simulink model "Wahsing_Mashine_1650800329"  (R2021a)
settings: Solver=VariableStepAuto  StartTime=0.0  StopTime=500  RelTol=1e-3
settings Model: Creator=Ish  LastModifiedBy=Ish

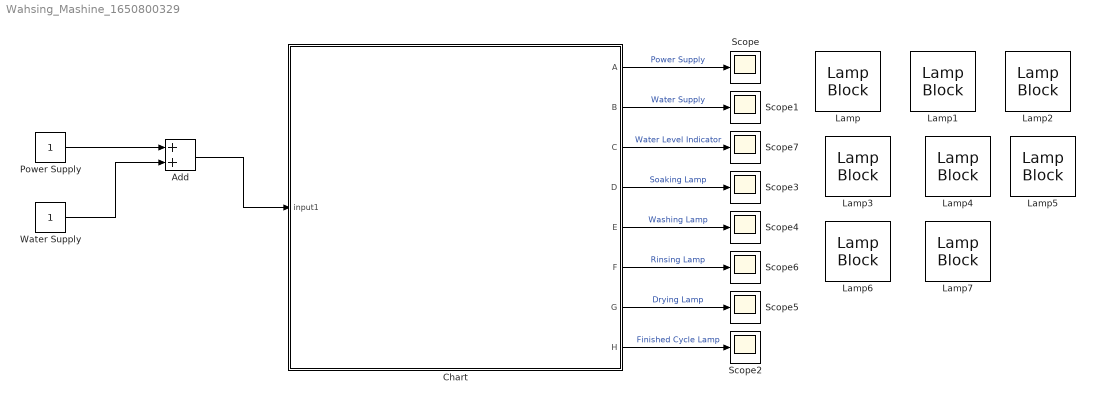
== system Wahsing_Mashine_1650800329 ==
  Add : Sum
  Chart : Stateflow chart  TreatAsAtomicUnit=on
  Lamp{,1..7} (8 alike) : LampBlock  Icon=Circle
  Power Supply : Constant
  Scope{,1..7} (8 alike) : Scope
  Water Supply : Constant
  wires:
  Water Supply/1 -> Add/2
  Power Supply/1 -> Add/1
  Add/1 -> Chart/1(input1)
  Chart/1(A) -> Scope/1  "Power Supply"
  Chart/2(B) -> Scope1/1  "Water Supply"
  Chart/3(C) -> Scope7/1  "Water Level Indicator"
  Chart/4(D) -> Scope3/1  "Soaking Lamp"
  Chart/5(E) -> Scope4/1  "Washing Lamp"
  Chart/6(F) -> Scope6/1  "Rinsing Lamp"
  Chart/7(G) -> Scope5/1  "Drying Lamp"
  Chart/8(H) -> Scope2/1  "Finished Cycle Lamp"

== stateflow chart Wahsing_Mashine_1650800329/Chart ==
  state State1
    entry:A=1,B=0
    exit:A=1,B=1
  state State2
    entry:A=1,B=1
    exit:B=1,C=0
  state State3
    entry:C=1,B=1,D=1
    exit:C=0,D=0
  state State4
    entry:D=0,E=1
    exit:E=0,F=1
  state State5
    entry:E=0,F=1
    exit:F=0,G=1
  state State6
    entry:F=0,G=1
    exit:G=0,H=1
  state State7
    entry:H=1
    exit:H=0
  (default) -> State1
  State1 -> State2 : [input1>1]
  State2 -> State1 [order 2] : [input1<1]
  State2 -> State3 [order 1] : [after(20,sec)]
  State3 -> State4 : [after(200,sec)]
  State4 -> State5 : [after(100,sec)]
  State5 -> State6 : [after(20,sec)]
  State6 -> State7 : [after(50,sec)]
  data: A output; B output; C output; D output; E output; F output; G output; H output; input1 input
